simulink model "Ex2_3"  (Simulink 6.0)
settings: Solver=FixedStepDiscrete  StartTime=0.0  StopTime=Tstop  FixedStep=1  RelTol=1e-3
values from neighbouring files (symbols this model uses):
  a = -0.01    [Ex2_1.m]    (also in Ex2_3launch.m = 0.001)
  Amp1 = 1    [Ex2_3launch.m]
  Amp2 = 1    [Ex2_3launch.m]
  infreq1 = 1169/(Tstop)    (= 0.0713065755764)    [Ex2_3launch.m]
  infreq2 = 1231/(Tstop)    (= 0.0750884469928)    [Ex2_3launch.m]
  N = 14    [Ex2_2launch.m]    (also in Ex2_3launch.m = 12)
  Npoint = 2^14+1    (= 16385)    [Ex2_2launch.m]    (also in Ex2_3launch.m = 16384)
libraries: simulink x1, dspsnks4 x1, dng_gmslib x1
settings Model: Creator=francomaloberti  LastModifiedBy=Cri  ExtModeAutoUpdateStatusClock=off
settings DataIOCC: SignalLoggingName=sigsOut
settings OptimizationCC: InlineInvariantSignals=off
settings DebuggingCC: SolverPrmCheckMsg=none
settings HardwareCC: TargetUnknown=on

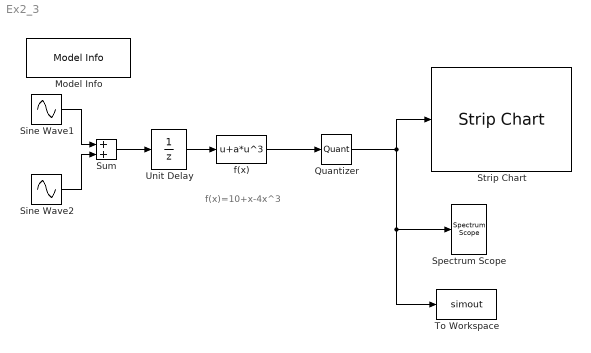
== system Ex2_3 ==
  note: f(x)=10+x-4x^3
  Model Info : simulink/Model-Wide Utilities/Model Info  InitialBlockCM=None  BlockCM=None  Frame=on  DisplayStringWithTags=Example 2.3 page 69  HorizontalTextAlignment=Center  LeftAlignmentValue=0.5  SourceBlockDiagram=Ex2_3  TagMaxNumber=20
  Quantizer : Quantizer  QuantizationInterval=1/2^N
  Sine Wave1 : Sin  Amplitude=Amp1  Frequency=2*pi*infreq1  SampleTime=0
  Sine Wave2 : Sin  Amplitude=Amp2  Frequency=2*pi*infreq2  SampleTime=0
  Spectrum Scope : dspsnks4/Spectrum Scope  ScopeProperties=on  Domain=Frequency  HorizSpan=1  UseBuffer=on  BufferSize=Npoint  Overlap=2  inpFftLenInherit=on  FFTlength=Npoint  numAvg=2^10  DisplayProperties=off  AxisGrid=on  Memory=on  FrameNumber=on  AxisLegend=off  AxisZoom=on  OpenScopeAtSimStart=off  OpenScopeImmediately=off  FigPos=[100 100 600 400]  AxisProperties=off  XUnits=Hertz  XRange=[0...Fs/2]  InheritXIncr=off  XIncr=1.0  XLabel=Samples  YUnits=dB  YLabel=Magnitude, dB  LineProperties=off  LineDisables=on  LineStyles=-  LineColors=[0 0 1]
      link override Periodogram: wintype=Blackman
      settings: YMin=-160  YMax=20
  Strip Chart : dng_gmslib/Strip Chart/Strip Chart  Tag=000  progid=mwStrip.stripctrl.1  connect=input  init="hActx.XTicMode = 1;hActx.XSpan = 10/60/60/24; hActx.TimeSecondsFormat = '%M:%S'; hActx.TimeDateFormat = ''; hActx.TimeDaysFormat = ''; hActx.TimeHoursFormat = ''; hActx.TimeMinutesFormat = ''; hActx.TimeMonthsFormat = ''; hActx.TimeYearsFormat = ''; % Set x-axis to display time; set span = 10 sec (in fixed units=days); set display format = \"min:sec\" only"  inblock=on  border=on  dialOut=0  updateParam=0
  Sum : Sum
  To Workspace : ToWorkspace  VariableName=simout  SampleTime=-1  SaveFormat=Array
  Unit Delay : UnitDelay
  "f(x) " : Fcn  Expr=u+a*u^3
  wires:
  Unit Delay/1 -> "f(x) "/1
  Quantizer/1 -> To Workspace/1, Spectrum Scope/1, Strip Chart/1
  Sum/1 -> Unit Delay/1
  Sine Wave1/1 -> Sum/1
  Sine Wave2/1 -> Sum/2
  "f(x) "/1 -> Quantizer/1
